simulink model "tp1_control2_simulink"  (R2021a)
settings: Solver=VariableStepAuto  StartTime=0.0  StopTime=500  RelTol=1e-3
libraries: cstblocks x5
settings Model: Creator=Pedro  LastModifiedBy=balta

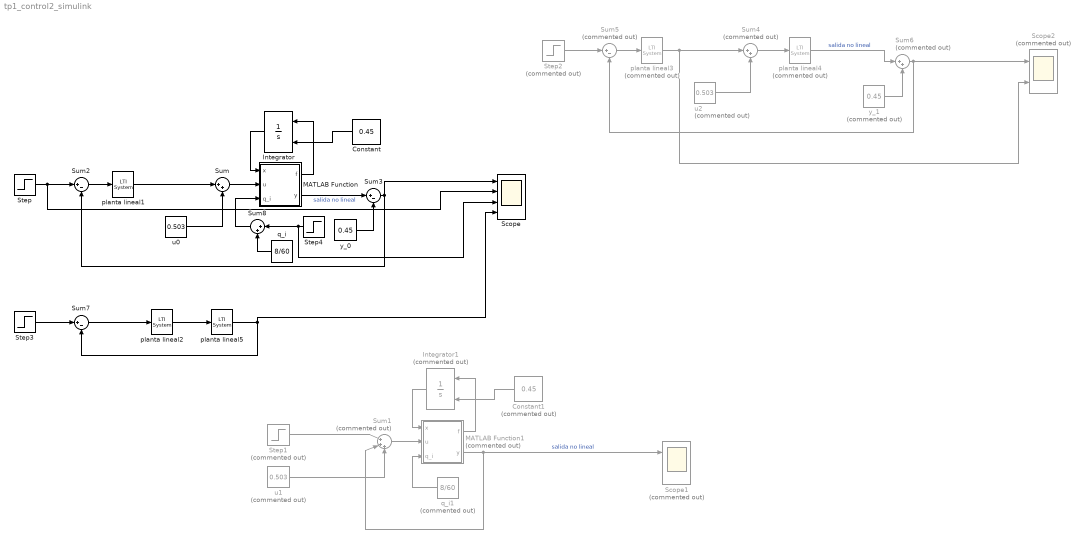
== system tp1_control2_simulink ==
  Constant : Constant  Value=0.45  VectorParams1D=off
  Constant1 : Constant  Commented=on  Value=0.45  VectorParams1D=off
  Integrator : Integrator  InitialConditionSource=external
  Integrator1 : Integrator  Commented=on  InitialConditionSource=external
  MATLAB Function : MATLAB Function  TreatAsAtomicUnit=on
  MATLAB Function1 : MATLAB Function  Commented=on  TreatAsAtomicUnit=on
  Scope : Scope  NumInputPorts=4
  Scope1 : Scope  Commented=on  NumInputPorts=2
  Scope2 : Scope  Commented=on  NumInputPorts=2
  Step : Step  Before=0.45  After=0.35  SampleTime=0
  Step1 : Step  Commented=on  Time=10  After=1.1 * 0.503  SampleTime=0
  Step2 : Step  Commented=on  Time=10  After=1.1 * 0.503  SampleTime=0
  Step3 : Step  Before=0.45  After=0.35  SampleTime=0
  Step4 : Step  Time=200  After=-8/600  SampleTime=0
  Sum : Sum  Inputs=|++
  Sum1 : Sum  Commented=on  Inputs=|+++
  Sum2 : Sum  Inputs=|+-
  Sum3 : Sum  Inputs=|+-
  Sum4 : Sum  Commented=on  Inputs=|++
  Sum5 : Sum  Commented=on  Inputs=|+-
  Sum6 : Sum  Commented=on  Inputs=|++
  Sum7 : Sum  Inputs=|+-
  Sum8 : Sum  Inputs=|++
  planta lineal1 : cstblocks/LTI System  sys=C_PI_Prima  IC=[]
  planta lineal2 : cstblocks/LTI System  sys=C_PI_Prima  IC=[]
  planta lineal3 : cstblocks/LTI System  Commented=on  sys=C_dig  IC=[]
  planta lineal4 : cstblocks/LTI System  Commented=on  sys=P_dis  IC=[]
  planta lineal5 : cstblocks/LTI System  sys=P_dis  IC=[]
  q_i : Constant  Value=8/60
  q_i1 : Constant  Commented=on  Value=8/60
  u0 : Constant  Value=0.503
  u1 : Constant  Commented=on  Value=0.503
  u2 : Constant  Commented=on  Value=0.503
  y_0 : Constant  Value=0.45
  y_1 : Constant  Commented=on  Value=0.45
  wires:
  MATLAB Function/1(f) -> Integrator/1
  Integrator/1 -> MATLAB Function/1(x)
  Constant/1 -> Integrator/2
  u0/1 -> Sum/2
  Sum/1 -> MATLAB Function/2(u)
  MATLAB Function/2(y) -> Sum3/1  "salida no lineal"
  y_0/1 -> Sum3/2
  Sum3/1 -> Sum2/2, Scope/1
  Step/1 -> Scope/2, Sum2/1
  Sum2/1 -> planta lineal1/1
  planta lineal1/1 -> Sum/1
  q_i1/1 -> MATLAB Function1/3(q_i)
  Sum1/1 -> MATLAB Function1/2(u)
  Step1/1 -> Sum1/1
  MATLAB Function1/1(f) -> Integrator1/1
  Integrator1/1 -> MATLAB Function1/1(x)
  Constant1/1 -> Integrator1/2
  MATLAB Function1/2(y) -> Scope1/1, Sum1/2  "salida no lineal"
  u1/1 -> Sum1/3
  Sum5/1 -> planta lineal3/1
  Sum4/1 -> planta lineal4/1
  Step2/1 -> Sum5/1
  Sum6/1 -> Sum5/2, Scope2/1
  planta lineal3/1 -> Scope2/2, Sum4/1
  y_1/1 -> Sum6/2
  u2/1 -> Sum4/2
  planta lineal4/1 -> Sum6/1  "salida no lineal"
  planta lineal2/1 -> planta lineal5/1
  planta lineal5/1 -> Sum7/2, Scope/4
  Sum7/1 -> planta lineal2/1
  Step3/1 -> Sum7/1
  Step4/1 -> Sum8/1, Scope/3
  q_i/1 -> Sum8/2
  Sum8/1 -> MATLAB Function/3(q_i)

== matlab function tp1_control2_simulink/MATLAB Function1 ==
  data: x input; u input; f output; y output; q_i input
function [f,y] = fcn(x,u,q_i)
d_2 = 10.65/1000 %metros diametro canio de salida
l_1 = 10/100%metros lado base inferior
l_2 = 40/100%metros lado base superior
l = 0.9%metros de la base del tanque al tope.
g = 9.81%metros/seg**2, gravedad Asumo que x1_punto eq = 0 (no hay variacion de altura)

f = ((q_i/1000 - (u*pi*(d_2^2/4)*(sqrt(2*g*x(1)))))/(l_1+(l_2-l_1)*(x(1)/l))^2);

y = x(1);

== matlab function tp1_control2_simulink/MATLAB Function ==
  data: x input; u input; f output; y output; q_i input
function [f,y] = fcn(x,u,q_i)
d_2 = 10.65/1000 %metros diametro canio de salida
l_1 = 10/100%metros lado base inferior
l_2 = 40/100%metros lado base superior
l = 0.9%metros de la base del tanque al tope.
g = 9.81%metros/seg**2, gravedad Asumo que x1_punto eq = 0 (no hay variacion de altura)

f = ((q_i/1000 - (u*pi*(d_2^2/4)*(sqrt(2*g*x(1)))))/(l_1+(l_2-l_1)*(x(1)/l))^2);

y = x(1);
